simulink model "hybrid_version"  (R2022a)
settings: Solver=VariableStepAuto  StartTime=0.0  StopTime=2  MaxStep=0.01  RelTol=1e-3
values from neighbouring files (symbols this model uses):
  k_gn = m*g/0.001    (= 412020)    [controller_parameters.m]
  k_gt = m*g/0.1    (= 4120.2)    [controller_parameters.m]
  m = 42    [controller_parameters.m]    (also in ground_reaction_params.m = 12)
  mu_slide = 0.8    [controller_parameters.m]    (also in ground_reaction_params.m = 0.008)
  mu_stick = 0.9    [controller_parameters.m]    (also in ground_reaction_params.m = 0.009)
  v_gn_max = 0.03    [controller_parameters.m]
  v_gt_max = 0.03    [controller_parameters.m]
  vLimit = 0.01    [controller_parameters.m]    (also in ground_reaction_params.m = 0.001)
undefined symbols (not defined in the file or in its folder): Newton, Raphson, X, Y, Z
libraries: sm_lib x179, nesl_utility x110, simulink x32, simulink_extras x8
(part 8 of 8)

== system hybrid_version/Bipedal Model with Torque Control/Right Ball C3/3D Contact/Kinetic Friction Model/Vector Norm ==
  vec : Inport
  Sqrt : Sqrt  OutputSignalType=real  AlgorithmType=Newton-Raphson
  Squares : Math  Operator=square  SignedPower=on  OutputSignalType=real
  Sum of Elements : Sum  Inputs=+
  norm : Outport
  wires:
  vec/1 -> Squares/1
  Sqrt/1 -> norm/1
  Sum of Elements/1 -> Sqrt/1
  Squares/1 -> Sum of Elements/1

== system hybrid_version/Bipedal Model with Torque Control/Right Ball C3/3D Contact/Static Friction Model/Vector Norm ==
  vec : Inport
  Sqrt : Sqrt  OutputSignalType=real  AlgorithmType=Newton-Raphson
  Squares : Math  Operator=square  SignedPower=on  OutputSignalType=real
  Sum of Elements : Sum  Inputs=+
  norm : Outport
  wires:
  vec/1 -> Squares/1
  Sqrt/1 -> norm/1
  Sum of Elements/1 -> Sqrt/1
  Squares/1 -> Sum of Elements/1

== system hybrid_version/Bipedal Model with Torque Control/Right Ball C4/3D Contact/Kinetic Friction Model/Vector Norm ==
  vec : Inport
  Sqrt : Sqrt  OutputSignalType=real  AlgorithmType=Newton-Raphson
  Squares : Math  Operator=square  SignedPower=on  OutputSignalType=real
  Sum of Elements : Sum  Inputs=+
  norm : Outport
  wires:
  Squares/1 -> Sum of Elements/1
  Sum of Elements/1 -> Sqrt/1
  Sqrt/1 -> norm/1
  vec/1 -> Squares/1

== system hybrid_version/Bipedal Model with Torque Control/Right Ball C4/3D Contact/Static Friction Model/Vector Norm ==
  vec : Inport
  Sqrt : Sqrt  OutputSignalType=real  AlgorithmType=Newton-Raphson
  Squares : Math  Operator=square  SignedPower=on  OutputSignalType=real
  Sum of Elements : Sum  Inputs=+
  norm : Outport
  wires:
  Squares/1 -> Sum of Elements/1
  Sum of Elements/1 -> Sqrt/1
  Sqrt/1 -> norm/1
  vec/1 -> Squares/1

== matlab function hybrid_version/ComputeCOP  ==
  data: right_foot_forces input; right_foot_contact input; left_foot_forces input; left_foot_contact input; left_x output; left_y output; right_x output; right_y output
function [left_x, left_y, right_x, right_y] = fcn(right_foot_forces, right_foot_contact, left_foot_forces, left_foot_contact)
    
    left_denom = (left_foot_forces(3)*left_foot_contact(1) + left_foot_forces(6)*left_foot_contact(2) + left_foot_forces(9)*left_foot_contact(3) + left_foot_forces(12)*left_foot_contact(4));
    left_y = ((-0.08*left_foot_forces(3)*left_foot_contact(1) - 0.08*left_foot_forces(6)*left_foot_contact(2)) + (0.0321*left_foot_forces(9)*left_foot_contact(3) + 0.0321*left_foot_forces(12)*left_foot_contact(4)))/left_denom;
    left_x = (0.02794*(left_foot_forces(3)*left_foot_contact(1) - left_foot_forces(6)*left_foot_contact(2) + left_foot_forces(9)*left_foot_contact(3) - left_foot_forces(12)*left_foot_contact(4)))/left_denom;


    right_denom = (right_foot_forces(3)*right_foot_contact(1) + right_foot_forces(6)*right_foot_contact(2) + right_foot_forces(9)*right_foot_contact(3) + right_foot_forces(12)*right_foot_contact(4));
    right_x = (0.02794*(right_foot_forces(3)*right_foot_contact(1) - right_foot_forces(6)*right_foot_contact(2) + right_foot_forces(9)*right_foot_contact(3) - right_foot_forces(12)*right_foot_contact(4)))/right_denom;
    right_y = ((-0.08*right_foot_forces(3)*right_foot_contact(1) -0.08*right_foot_forces(6)*right_foot_contact(2)) + (0.0321*right_foot_forces(9)*right_foot_contact(3) + 0.0321*right_foot_forces(12)*right_foot_contact(4)))/right_denom;

end
